simulink subsystem "MyPieroSensoresDistancia"  (R2022b)
settings: Solver=VariableStepAuto  StartTime=0.0  StopTime=10.0  RelTol=1e-3
settings Model: Creator=Usuario  LastModifiedBy=Usuario

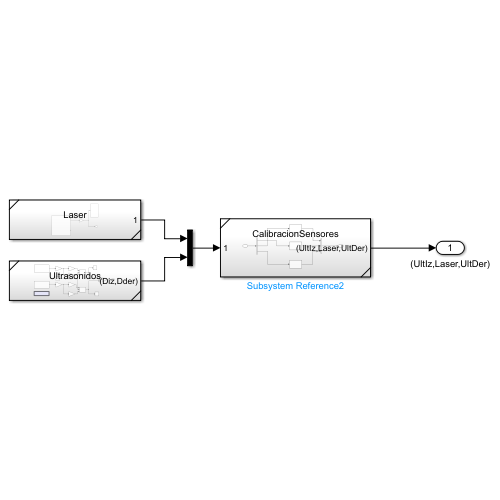
[thumbnail: Simulink's stored preview of the top-level diagram]
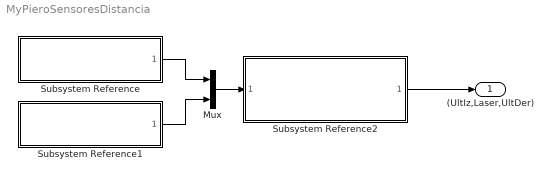
== system MyPieroSensoresDistancia ==
  Mux : Mux  Inputs=2
  Subsystem Reference : Subsystem  ReferencedSubsystem=Laser
  Subsystem Reference1 : Subsystem  ReferencedSubsystem=Ultrasonidos
  Subsystem Reference2 : Subsystem  ReferencedSubsystem=CalibracionSensores
  (UltIz,Laser,UltDer) : Outport
  wires:
  Subsystem Reference1/1 -> Mux/2
  Subsystem Reference/1 -> Mux/1
  Subsystem Reference2/1 -> (UltIz,Laser,UltDer)/1
  Mux/1 -> Subsystem Reference2/1
